simulink model "heli_q8_oppgave1"  (R2020b)
settings: Solver=ode1  StartTime=0.0  StopTime=50  FixedStep=0.002  RelTol=1e-3  EnableMultiTasking=on
PostLoadFcn:
  | qc_set_target_type(getConfigSet(bdroot, 'QUARC Default Target Configuration'));
values from neighbouring files (symbols this model uses):
  A = [0 1 0; 0 0 0; 0 0 0]    [init_heli_1_2.m]
  B = [0 0; 0 k_1; k_2 0]    [init_heli_1_2.m]
  C = [1 0 0; 0 0 1]    [init_heli_1_2.m]
  F = (C*(B*K-A)^-1*B)^-1    [init_heli_1_2.m]
  Joystick_gain_x = 1    [init_heli_1_2.m]
  Joystick_gain_y = -1    [init_heli_1_2.m]
  Vs_0 = 6    [init_heli_1_2.m]
undefined symbols (not defined in the file or in its folder): HIL, K, qc_get_step_size
libraries: quarc_library x4
settings Model: SimulationMode=external  ExtModeTrigDuration=60000  Creator=Rchan  LastModifiedBy=pederhly
settings SolverCC: PositivePriorityOrder=on
settings DataIOCC: LimitDataPoints=on  SaveFormat=Array  SignalLoggingSaveFormat=ModelDataLogs  ReturnWorkspaceOutputs=off
settings OptimizationCC: ExpressionDepthLimit=2147483647  InitFltsAndDblsToZero=on  LifeSpan=inf
settings DebuggingCC: SaveWithParameterizedLinksMsg=none  UnderspecifiedInitializationDetection=Classic  MergeDetectMultiDrivingBlocksExec=none  SolverPrmCheckMsg=warning  MultiTaskDSMMsg=warning  MultiTaskCondExecSysMsg=none  FcnCallInpInsideContextMsg=warning  AllowSymbolicDim=off  StateNameClashWarn=warning  SFUnexpectedBacktrackingDiag=warning  SFNoUnconditionalDefaultTransitionDiag=warning  SFExecutionAtInitializationDiag=none  ArithmeticOperatorsInVariantConditions=warning
settings HardwareCC: ProdBitPerPointer=32  ProdBitPerSizeT=32  ProdBitPerPtrDiffT=32  ProdLargestAtomicFloat=None  ProdIntDivRoundTo=Undefined  ProdEndianess=Unspecified  ProdWordSize=32  ProdHWDeviceType=32-bit Generic
settings ModelReferenceCC: PropagateSignalLabelsOutOfModel=off
settings SFSimCC: SimUseLocalCustomCode=off  CustomCodeUndefinedFunction=UseInterfaceOnly
settings RTWCC: Description=QUARC Win64 Target  SystemTargetFile=quarc_win64.tlc  TemplateMakefile=quarc_default_tmf  RTWUseLocalCustomCode=off
settings CodeAppCC: StateflowObjectComments=on
settings GRTTargetCC: TargetLangStandard=C89/C90 (ANSI)  ParMdlRefBuildCompliant=off  CompOptLevelCompliant=off  CombineOutputUpdateFcns=off  MatFileLogging=off  GRTInterface=on  UseToolchainInfoCompliant=off  ExtMode=on  ExtModeMexFile=quarc_comm
settings ConfigComp: CovMetricSettings=dw  CovSaveCumulativeToWorkspaceVar=on  CovSaveSingleToWorkspaceVar=on  CovExternalEMLEnable=off  CovSFcnEnable=off

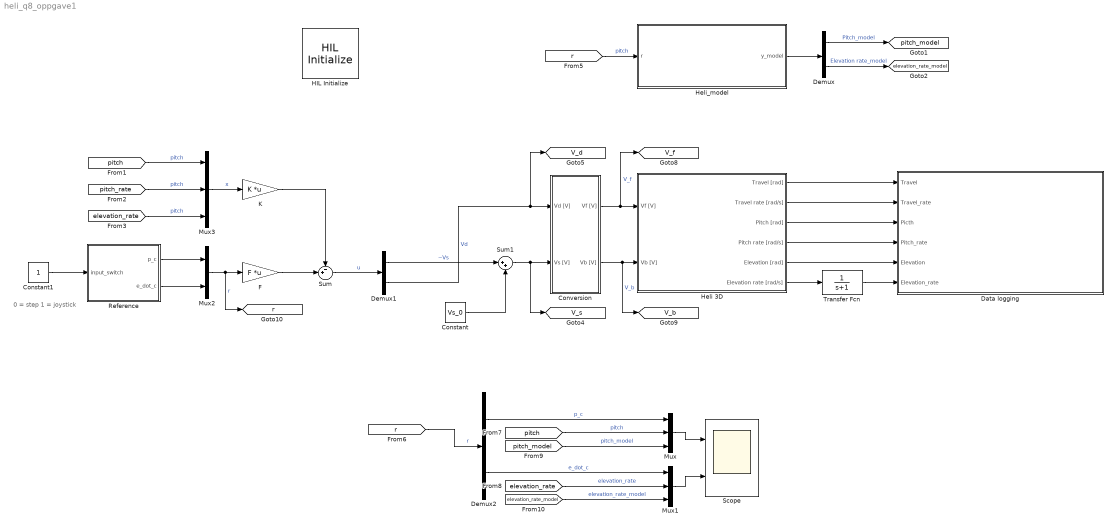
== system heli_q8_oppgave1 ==
  note: 0 = step
      | 1 = joystick
  Constant : Constant  Value=Vs_0
  Constant1 : Constant
  Conversion : Subsystem
  Data logging : Subsystem
  Demux : Demux  Outputs=2
  Demux1 : Demux  Outputs=2
  Demux2 : Demux  Outputs=2
  F : Gain  Gain=F  Multiplication=Matrix(K*u) (u vector)
  HIL Initialize : quarc_library/Data Acquisition/Generic/Configuration/HIL Initialize  Priority=-99  object_name=HIL-1  board_type=q8_usb  board_number=0  board_options=update_rate=normal;decimation=1  exclusive=off  active=off  hardware_clocks=[0:2]  clock_modes=[]  initial_clock_frequencies=[]  set_clock_params_at_start=off  set_clock_params_at_switch_in=off  set_clock_frequencies_at_start=off  set_clock_frequencies_at_switch_in=off  analog_input_channels=[0:7]  analog_input_configurations=[]  analog_input_maximums=10  analog_input_minimums=-10  set_analog_input_params_at_start=on  set_analog_input_params_at_switch_in=off  analog_output_channels=[0:7]  analog_output_maximums=10  analog_output_minimums=-10  initial_analog_outputs=[0]  final_analog_outputs=[0]  watchdog_analog_outputs=0  set_analog_output_params_at_start=on  set_analog_output_params_at_switch_in=off  set_analog_outputs_at_start=on  set_analog_outputs_at_switch_in=off  set_analog_outputs_at_terminate=on  set_analog_outputs_at_switch_out=off  set_analog_outputs_on_watchdog=off  digital_input_channels=[]  digital_output_channels=[]  digital_output_configuration=[]  initial_digital_outputs=[1]  final_digital_outputs=[1]  watchdog_digital_outputs=[1]  set_digital_output_params_at_start=off  set_digital_output_params_at_switch_in=off  set_digital_outputs_at_start=on  set_digital_outputs_at_switch_in=off  set_digital_outputs_at_terminate=on  set_digital_outputs_at_switch_out=off  set_digital_outputs_on_watchdog=off  encoder_channels=[0:7]  quadrature=[4]  encoder_filter_frequency=[]  initial_encoder_counts=[0]  set_encoder_params_at_start=on  set_encoder_params_at_switch_in=off  set_encoder_counts_at_start=on  set_encoder_counts_at_switch_in=off  pwm_channels=[0:7]  pwm_modes=0  pwm_frequency=99.532799999999995e6/4095  pwm_configuration=[0]  pwm_alignment=[0]  pwm_polarity=[1]  pwm_leading_deadband=[0]  pwm_trailing_deadband=[0]  initial_pwm_outputs=[0]  final_pwm_outputs=[0]  watchdog_pwm_outputs=[0]  set_pwm_params_at_start=on  set_pwm_params_at_switch_in=off  set_pwm_outputs_at_start=on  set_pwm_outputs_at_switch_in=off  set_pwm_outputs_at_terminate=on  set_pwm_outputs_at_switch_out=off  set_pwm_outputs_on_watchdog=off  other_output_channels=[]  initial_other_outputs=[]  final_other_outputs=[]  watchdog_other_outputs=[]  set_other_outputs_at_start=off  set_other_outputs_at_switch_in=off  set_other_outputs_at_terminate=off  set_other_outputs_at_switch_out=off  set_other_outputs_on_watchdog=off
  Heli 3D : Subsystem
  Heli_model : Subsystem
  K : Gain  Gain=K  Multiplication=Matrix(K*u) (u vector)
  Mux : Mux  Inputs=3
  Mux1 : Mux  Inputs=3
  Mux2 : Mux  Inputs=2
  Mux3 : Mux  Inputs=3
  Reference : Subsystem
  Scope : Scope  NumInputPorts=2
  Sum : Sum  Inputs=-+|
  Sum1 : Sum  Inputs=|++
  Transfer Fcn : TransferFcn  Denominator=[1 1]
  tag scope: V_b=global, V_d=global, V_f=global, V_s=global, elevation_rate_model=global, pitch_model=global, r=global
  wires:
  Conversion/2(Vb [V]) -> [V_b], Heli 3D/2(Vb [V])  "V_b"
  Conversion/1(Vf [V]) -> [V_f], Heli 3D/1(Vf [V])  "V_f"
  [pitch] -> Mux3/1  "pitch"
  [pitch_rate] -> Mux3/2  "pitch"
  [elevation_rate] -> Mux3/3  "pitch"
  Mux3/1 -> K/1  "x"
  Mux2/1 -> [r], F/1  "r"
  F/1 -> Sum/2
  K/1 -> Sum/1
  Sum/1 -> Demux1/1  "u"
  Demux1/2 -> [V_d], Conversion/1(Vd [V])  "Vd"
  Sum1/1 -> [V_s], Conversion/2(Vs [V])
  Constant/1 -> Sum1/2
  Demux1/1 -> Sum1/1  "~Vs"
  Demux/1 -> [pitch_model]  "Pitch_model"
  Demux/2 -> [elevation_rate_model]  "Elevation rate_model"
  Heli_model/1(y_model) -> Demux/1
  Heli 3D/1(Travel [rad]) -> Data logging/1(Travel)
  Heli 3D/3(Pitch [rad]) -> Data logging/3(Picth)
  Heli 3D/2(Travel rate [rad/s]) -> Data logging/2(Travel_rate)
  Heli 3D/4(Pitch rate [rad/s]) -> Data logging/4(Pitch_rate)
  Heli 3D/5(Elevation [rad]) -> Data logging/5(Elevation)
  Reference/1(p_c) -> Mux2/1
  Reference/2(e_dot_c) -> Mux2/2
  Constant1/1 -> Reference/1(input_switch)
  [r] -> Demux2/1  "r"
  Demux2/1 -> Mux/1  "p_c"
  [pitch] -> Mux/2  "pitch"
  Demux2/2 -> Mux1/1  "e_dot_c"
  [elevation_rate] -> Mux1/2  "elevation_rate"
  Mux/1 -> Scope/1
  Mux1/1 -> Scope/2
  [r] -> Heli_model/1(r)  "pitch"
  Heli 3D/6(Elevation rate [rad/s]) -> Transfer Fcn/1
  Transfer Fcn/1 -> Data logging/6(Elevation_rate)
  [pitch_model] -> Mux/3  "pitch_model"
  [elevation_rate_model] -> Mux1/3  "elevation_rate_model"

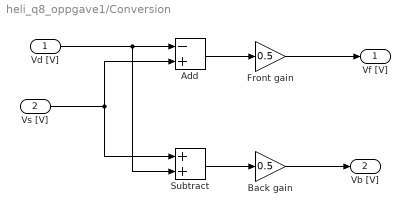
== system heli_q8_oppgave1/Conversion ==
  Vd [V] : Inport
  Vs [V] : Inport  Port=2
  Add : Sum  Inputs=-+
  Back gain : Gain  Gain=0.5
  Front gain : Gain  Gain=0.5
  Subtract : Sum
  Vf [V] : Outport
  Vb [V] : Outport  Port=2
  wires:
  Vd [V]/1 -> Subtract/2, Add/1
  Vs [V]/1 -> Subtract/1, Add/2
  Subtract/1 -> Back gain/1
  Back gain/1 -> Vb [V]/1
  Add/1 -> Front gain/1
  Front gain/1 -> Vf [V]/1

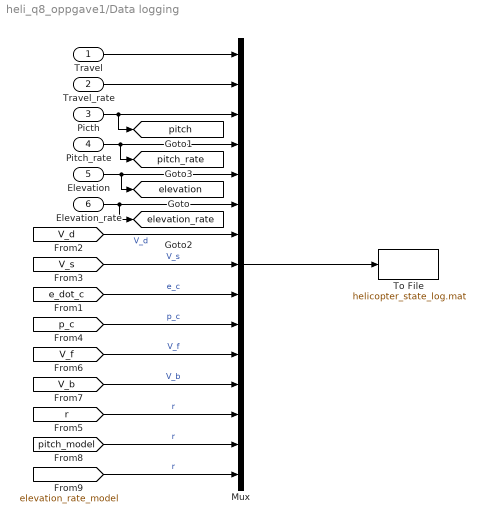
== system heli_q8_oppgave1/Data logging ==
  Travel : Inport
  Travel_rate : Inport  Port=2
  Picth : Inport  Port=3
  Pitch_rate : Inport  Port=4
  Elevation : Inport  Port=5
  Elevation_rate : Inport  Port=6
  Mux : Mux  Inputs=15
  To File : ToFile  Filename=helicopter_state_log.mat  MatrixName=var
  tag scope: elevation=global, elevation_rate=global, pitch=global, pitch_rate=global
  wires:
  Pitch_rate/1 -> [pitch_rate], Mux/4
  Elevation/1 -> [elevation], Mux/5
  Travel/1 -> Mux/1
  Travel_rate/1 -> Mux/2
  Mux/1 -> To File/1
  Elevation_rate/1 -> [elevation_rate], Mux/6
  Picth/1 -> [pitch], Mux/3
  [V_s] -> Mux/8  "V_s"
  [V_b] -> Mux/12  "V_b"
  [p_c] -> Mux/10  "p_c"
  [e_dot_c] -> Mux/9  "e_c"
  [V_d] -> Mux/7  "V_d"
  [V_f] -> Mux/11  "V_f"
  [r] -> Mux/13  "r"
  [pitch_model] -> Mux/14  "r"
  [elevation_rate_model] -> Mux/15  "r"

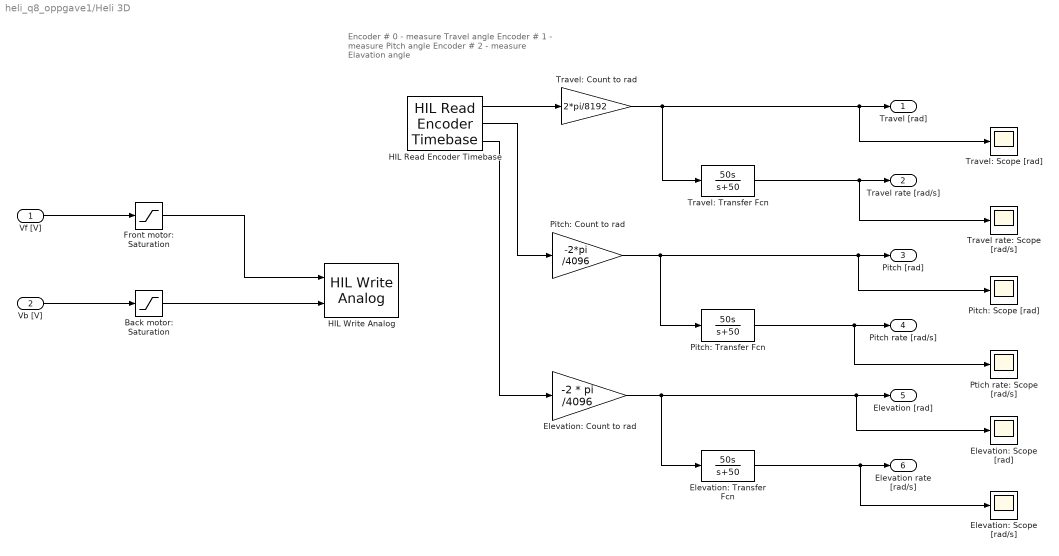
== system heli_q8_oppgave1/Heli 3D ==
  note: Encoder # 0 - measure Travel angle
      | Encoder # 1 - measure Pitch angle
      | Encoder # 2 - measure Elavation angle
  Vf [V] : Inport
  Vb [V] : Inport  Port=2
  Back motor: Saturation : Saturate  UpperLimit=5  LowerLimit=-5
  Elevation: Count to rad : Gain  Gain=-2 * pi /4096
  Elevation: Scope [rad/s] : Scope
  Elevation: Scope [rad] : Scope
  Elevation: Transfer Fcn : TransferFcn  Numerator=[50 0]  Denominator=[1 50]
  Front motor: Saturation : Saturate  UpperLimit=5  LowerLimit=-5
  HIL Read Encoder Timebase : quarc_library/Data Acquisition/Generic/Timebases/HIL Read Encoder Timebase  object_name=HIL-1  clock=0  channels=[0:2]  active=on  vector_output=off  data_type_mode=Inherit via back propagation  data_type=double  overflow_mode=Error on overflow  samples_in_buffer=max(ceil(1/qc_get_step_size), 1)
  HIL Write Analog : quarc_library/Data Acquisition/Generic/Immediate I//O/HIL Write Analog  object_name=HIL-1  channels=[0:1]  sample_time=-1  active=off  vector_input=off
  Pitch: Count to rad : Gain  Gain=-2*pi /4096
  Pitch: Scope [rad] : Scope
  Pitch: Transfer Fcn : TransferFcn  Numerator=[50 0]  Denominator=[1 50]
  Ptich rate: Scope [rad/s] : Scope
  Travel rate: Scope [rad/s] : Scope
  Travel: Count to rad : Gain  Gain=2*pi/8192
  Travel: Scope [rad] : Scope
  Travel: Transfer Fcn : TransferFcn  Numerator=[50 0]  Denominator=[1 50]
  Travel [rad] : Outport
  Travel rate [rad/s] : Outport  Port=2
  Pitch [rad] : Outport  Port=3
  Pitch rate [rad/s] : Outport  Port=4
  Elevation [rad] : Outport  Port=5
  Elevation rate [rad/s] : Outport  Port=6
  wires:
  HIL Read Encoder Timebase/1 -> Travel: Count to rad/1
  HIL Read Encoder Timebase/2 -> Pitch: Count to rad/1
  HIL Read Encoder Timebase/3 -> Elevation: Count to rad/1
  Travel: Count to rad/1 -> Travel: Scope [rad]/1, Travel [rad]/1, Travel: Transfer Fcn/1
  Travel: Transfer Fcn/1 -> Travel rate: Scope [rad/s]/1, Travel rate [rad/s]/1
  Pitch: Count to rad/1 -> Pitch: Transfer Fcn/1, Pitch: Scope [rad]/1, Pitch [rad]/1
  Pitch: Transfer Fcn/1 -> Ptich rate: Scope [rad/s]/1, Pitch rate [rad/s]/1
  Elevation: Count to rad/1 -> Elevation: Transfer Fcn/1, Elevation: Scope [rad]/1, Elevation [rad]/1
  Elevation: Transfer Fcn/1 -> Elevation: Scope [rad/s]/1, Elevation rate [rad/s]/1
  Vf [V]/1 -> Front motor: Saturation/1
  Vb [V]/1 -> Back motor: Saturation/1
  Front motor: Saturation/1 -> HIL Write Analog/1
  Back motor: Saturation/1 -> HIL Write Analog/2

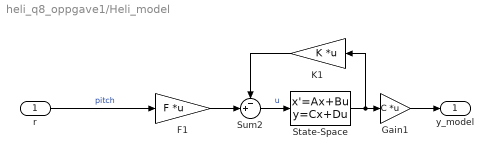
== system heli_q8_oppgave1/Heli_model ==
  r : Inport
  F1 : Gain  Gain=F  Multiplication=Matrix(K*u) (u vector)
  Gain1 : Gain  Gain=C  Multiplication=Matrix(K*u) (u vector)
  K1 : Gain  Gain=K  Multiplication=Matrix(K*u) (u vector)
  State-Space : StateSpace  A=A  B=B  C=eye(3)  D=[0 0; 0 0; 0 0]  InitialCondition=0
  Sum2 : Sum  Inputs=-+|
  y_model : Outport
  wires:
  Gain1/1 -> y_model/1
  F1/1 -> Sum2/2
  r/1 -> F1/1  "pitch"
  Sum2/1 -> State-Space/1  "u"
  State-Space/1 -> K1/1, Gain1/1
  K1/1 -> Sum2/1

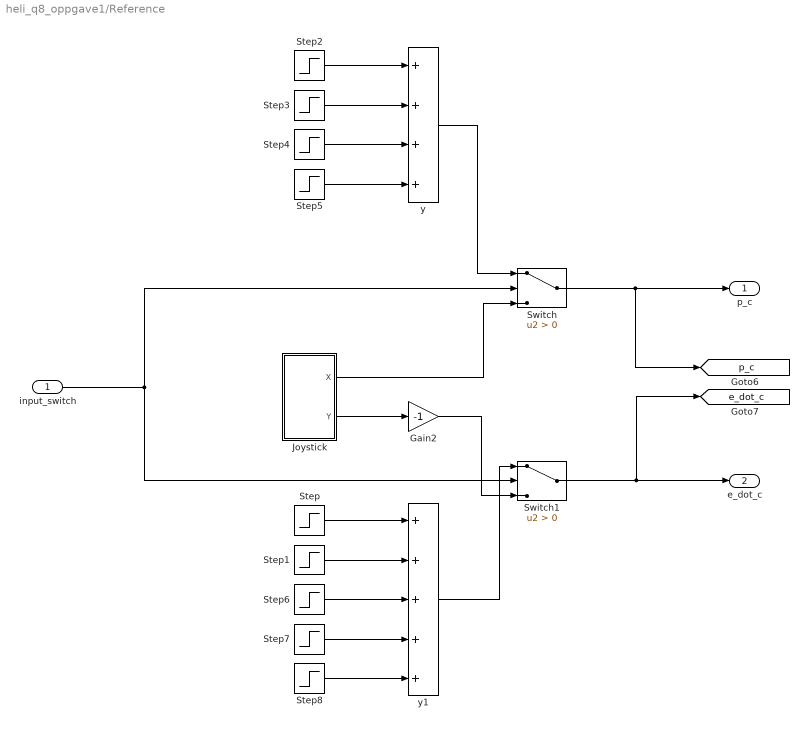
== system heli_q8_oppgave1/Reference ==
  input_switch : Inport
  Gain2 : Gain  Gain=-1
  Joystick : Subsystem
  Step : Step  Time=10  After=0.1  SampleTime=0
  Step1 : Step  Time=15  After=-0.2  SampleTime=0
  Step2 : Step  Time=25  After=0.5  SampleTime=0
  Step3 : Step  Time=35  After=-0.5  SampleTime=0
  Step4 : Step  Time=40  After=0.7  SampleTime=0
  Step5 : Step  Time=45  After=-0.7  SampleTime=0
  Step6 : Step  Time=20  After=0.1  SampleTime=0
  Step7 : Step  Time=40  After=0.1  SampleTime=0
  Step8 : Step  Time=45  After=-0.1  SampleTime=0
  Switch : Switch  Criteria=u2 > Threshold
  Switch1 : Switch  Criteria=u2 > Threshold
  y : Sum  Inputs=++++
  y1 : Sum  Inputs=+++++
  p_c : Outport
  e_dot_c : Outport  Port=2
  tag scope: e_dot_c=global, p_c=global
  wires:
  y1/1 -> Switch1/1
  y/1 -> Switch/1
  input_switch/1 -> Switch1/2, Switch/2
  Switch/1 -> [p_c], p_c/1
  Joystick/1(X) -> Switch/3
  Switch1/1 -> [e_dot_c], e_dot_c/1
  Joystick/2(Y) -> Gain2/1
  Step/1 -> y1/1
  Step3/1 -> y/2
  Step2/1 -> y/1
  Gain2/1 -> Switch1/3
  Step4/1 -> y/3
  Step5/1 -> y/4
  Step1/1 -> y1/2
  Step7/1 -> y1/4
  Step6/1 -> y1/3
  Step8/1 -> y1/5

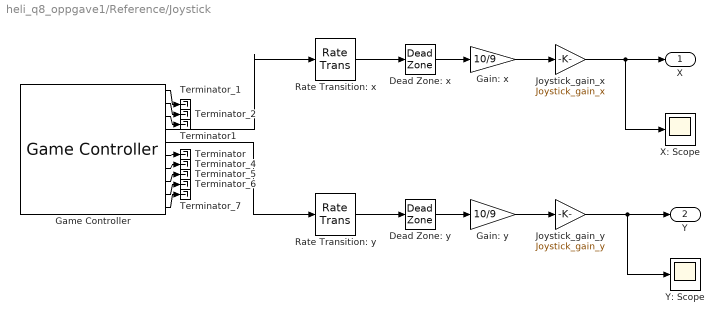
== system heli_q8_oppgave1/Reference/Joystick ==
  Dead Zone: x : DeadZone  LowerValue=-0.1  UpperValue=0.1  SaturateOnIntegerOverflow=on
  Dead Zone: y : DeadZone  LowerValue=-0.1  UpperValue=0.1  SaturateOnIntegerOverflow=on
  Gain: x : Gain  Gain=10/9
  Gain: y : Gain  Gain=10/9
  Game Controller : quarc_library/Devices/Peripherals/Target/Game Controller  controller=1  buffer_size=12  deadzone=[]  saturation=[]  sample_time=max(qc_get_step_size, 0.01)  auto_center=off  enabled=on
      settings: SourceProductName=QUARC Targets
  Joystick_gain_x : Gain  Gain=Joystick_gain_x
  Joystick_gain_y : Gain  Gain=Joystick_gain_y
  Rate Transition: x : RateTransition
  Rate Transition: y : RateTransition
  Terminator : Terminator
  Terminator1 : Terminator
  Terminator_{1..2,4..7} (6 alike) : Terminator
  X: Scope : Scope
  Y: Scope : Scope
  X : Outport
  Y : Outport  Port=2
  wires:
  Rate Transition: y/1 -> Dead Zone: y/1
  Rate Transition: x/1 -> Dead Zone: x/1
  Game Controller/5 -> Rate Transition: y/1
  Game Controller/4 -> Rate Transition: x/1
  Game Controller/1 -> Terminator_1/1
  Game Controller/2 -> Terminator_2/1
  Game Controller/7 -> Terminator_4/1
  Game Controller/8 -> Terminator_5/1
  Game Controller/9 -> Terminator_6/1
  Game Controller/10 -> Terminator_7/1
  Game Controller/3 -> Terminator1/1
  Game Controller/6 -> Terminator/1
  Dead Zone: x/1 -> Gain: x/1
  Dead Zone: y/1 -> Gain: y/1
  Gain: x/1 -> Joystick_gain_x/1
  Gain: y/1 -> Joystick_gain_y/1
  Joystick_gain_x/1 -> X/1, X: Scope/1
  Joystick_gain_y/1 -> Y: Scope/1, Y/1
